simulink model "ObservadorPlantaBuenazo"  (R2016a)
settings: Solver=ode45  StartTime=0.0  StopTime=10  MaxStep=0.01  RelTol=1e-3
settings Model: Creator=i95sa  LastModifiedBy=i95sa
settings DataIOCC: SaveFormat=StructureWithTime
settings DebuggingCC: FcnCallInpInsideContextMsg=EnableAllAsWarning
settings HardwareCC: ProdWordSize=32  ProdHWDeviceType=Specified
settings ConfigComp: CovSFcnEnable=off

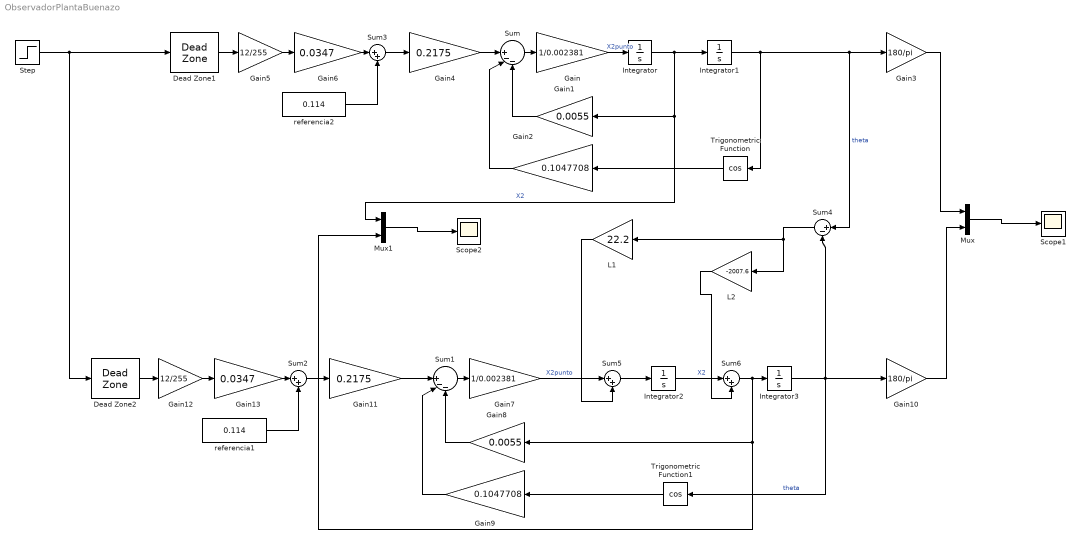
== system ObservadorPlantaBuenazo ==
  Dead Zone1 : DeadZone  LowerValue=0  UpperValue=0  SaturateOnIntegerOverflow=on
  Dead Zone2 : DeadZone  LowerValue=0  UpperValue=0  SaturateOnIntegerOverflow=on
  Gain : Gain  Gain=1/0.002381
  Gain1 : Gain  Gain=0.0055
  Gain10 : Gain  Gain=180/pi
  Gain11 : Gain  Gain=0.2175
  Gain12 : Gain  Gain=12/255
  Gain13 : Gain  Gain=0.0347
  Gain2 : Gain  Gain=0.1047708
  Gain3 : Gain  Gain=180/pi
  Gain4 : Gain  Gain=0.2175
  Gain5 : Gain  Gain=12/255
  Gain6 : Gain  Gain=0.0347
  Gain7 : Gain  Gain=1/0.002381
  Gain8 : Gain  Gain=0.0055
  Gain9 : Gain  Gain=0.1047708
  Integrator : Integrator
  Integrator1 : Integrator  InitialCondition=-0.65
  Integrator2 : Integrator
  Integrator3 : Integrator  InitialCondition=-0.65
  L1 : Gain  Gain=22.2
  L2 : Gain  Gain=-2007.6
  Mux : Mux  Inputs=2
  Mux1 : Mux  Inputs=2
  Scope1 : Scope
  Scope2 : Scope
  Step : Step  Time=0  After=221  SampleTime=0
  Sum : Sum  Inputs=||+--
  Sum1 : Sum  Inputs=||+--
  Sum{2..3,5..6} (4 alike) : Sum  Inputs=|++
  Sum4 : Sum  Inputs=|+-
  Trigonometric Function : Trigonometry  Operator=cos
  Trigonometric Function1 : Trigonometry  Operator=cos
  referencia1 : Constant  Value=0.114
  referencia2 : Constant  Value=0.114
  wires:
  Sum/1 -> Gain/1
  Gain/1 -> Integrator/1  "X2punto"
  Integrator/1 -> Mux1/1, Gain1/1, Integrator1/1  "X2"
  Trigonometric Function/1 -> Gain2/1
  Gain1/1 -> Sum/3
  Integrator1/1 -> Sum4/1, Gain3/1, Trigonometric Function/1  "theta"
  Gain2/1 -> Sum/2
  Gain4/1 -> Sum/1
  referencia2/1 -> Sum3/2
  Sum3/1 -> Gain4/1
  Gain5/1 -> Gain6/1
  Gain6/1 -> Sum3/1
  Dead Zone1/1 -> Gain5/1
  Sum1/1 -> Gain7/1
  Integrator2/1 -> Sum6/1  "X2"
  Trigonometric Function1/1 -> Gain9/1
  Gain8/1 -> Sum1/3
  Integrator3/1 -> Sum4/2, Trigonometric Function1/1, Gain10/1  "theta"
  Gain9/1 -> Sum1/2
  Gain11/1 -> Sum1/1
  referencia1/1 -> Sum2/2
  Sum2/1 -> Gain11/1
  Gain12/1 -> Gain13/1
  Gain13/1 -> Sum2/1
  Dead Zone2/1 -> Gain12/1
  Step/1 -> Dead Zone1/1, Dead Zone2/1
  Gain7/1 -> Sum5/1  "X2punto"
  Sum5/1 -> Integrator2/1
  Sum4/1 -> L2/1, L1/1
  Sum6/1 -> Mux1/2, Gain8/1, Integrator3/1
  L2/1 -> Sum6/2
  L1/1 -> Sum5/2
  Gain3/1 -> Mux/1
  Mux/1 -> Scope1/1
  Gain10/1 -> Mux/2
  Mux1/1 -> Scope2/1
